simulink model "LinearesSystem"  (R2021b)
settings: Solver=ode4  StartTime=0.0  StopTime=50  FixedStep=0.02  RelTol=1e-3
undefined symbols (not defined in the file): BFZ, ENV
settings Model: Creator=jonih  LastModifiedBy=jonih

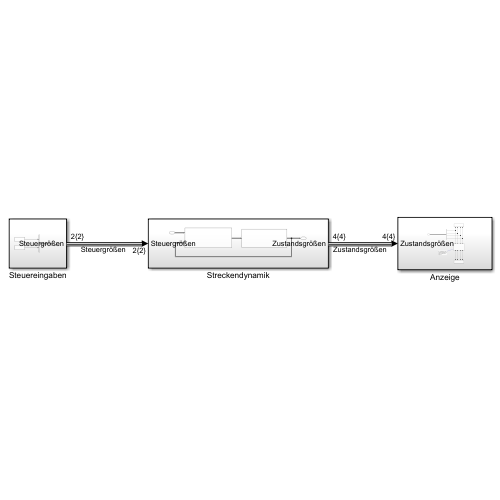
[thumbnail: Simulink's stored preview of the top-level diagram]
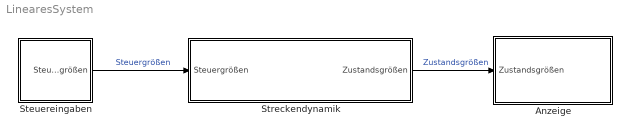
== system LinearesSystem ==
  Anzeige : Subsystem
  Steuereingaben : Subsystem
  Streckendynamik : Subsystem
  wires:
  Steuereingaben/1(Steuergrößen) -> Streckendynamik/1(Steuergrößen)  "Steuergrößen"
  Streckendynamik/1(Zustandsgrößen) -> Anzeige/1(Zustandsgrößen)  "Zustandsgrößen"

== system LinearesSystem/Anzeige ==
  note: zur Herstellung der
      | Vergleichbarkeit mit
      | dem nichtlinearen
      | System
  Zustandsgrößen : Inport
  Aufaddierung der Initalwerte : Subsystem
  Bus Selector : BusSelector  OutputSignals=ΔV,Δγ,Δq,Δα
  lineares System : Scope  NumInputPorts=4
  lineares System (angepasst) : Scope  NumInputPorts=4
  wires:
  Zustandsgrößen/1 -> Bus Selector/1  "Abweichung Zust. vom BFZ"
  Bus Selector/1 -> Aufaddierung der Initalwerte/1(<ΔV>), lineares System/1  "<ΔV>"
  Bus Selector/2 -> Aufaddierung der Initalwerte/2(<Δγ>), lineares System/2  "<Δγ>"
  Bus Selector/3 -> lineares System/3, Aufaddierung der Initalwerte/3(<Δq>)  "<Δq>"
  Bus Selector/4 -> lineares System/4, Aufaddierung der Initalwerte/4(<Δα>)  "<Δα>"
  Aufaddierung der Initalwerte/1(V) -> lineares System (angepasst)/1  "V"
  Aufaddierung der Initalwerte/2(gamma) -> lineares System (angepasst)/2  "gamma"
  Aufaddierung der Initalwerte/3(q) -> lineares System (angepasst)/3  "q"
  Aufaddierung der Initalwerte/4(alpha) -> lineares System (angepasst)/4  "alpha"

== system LinearesSystem/Steuereingaben ==
  Bus Creator : BusCreator  Inputs=2
  Δδ : Constant  Value=0
  Δη : Constant  Value=0
  Steuergrößen : Outport
  wires:
  Δη/1 -> Bus Creator/1  "Δη"
  Δδ/1 -> Bus Creator/2  "Δδ"
  Bus Creator/1 -> Steuergrößen/1  "Steuergrößen"

== system LinearesSystem/Streckendynamik ==
  Steuergrößen : Inport
  Berechnung Änderung der Zustandsgrößen : Subsystem
  Integration : Subsystem
  Zustandsgrößen : Outport
  wires:
  Berechnung Änderung der Zustandsgrößen/1(zeitliche Änderung der Zustandsgrößen) -> Integration/1(zeitliche Änderung der Zustandsgrößen)
  Integration/1(Zustandsgrößen) -> Berechnung Änderung der Zustandsgrößen/2(Zustandsgrößen), Zustandsgrößen/1  "Zustandsgrößen"
  Steuergrößen/1 -> Berechnung Änderung der Zustandsgrößen/1(Steuergrößen)

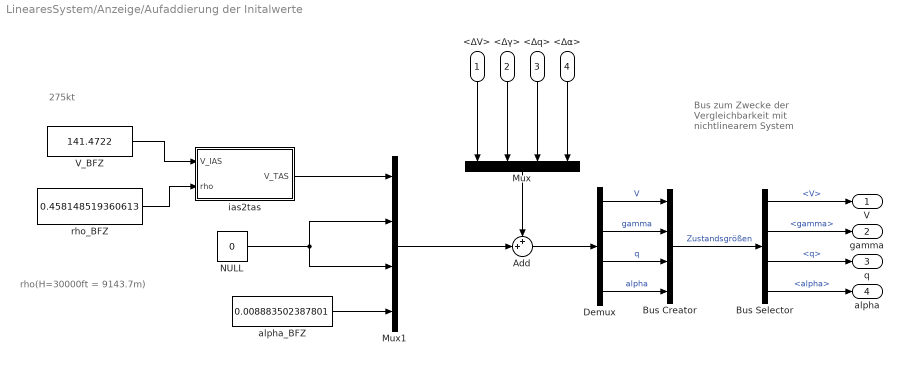
== system LinearesSystem/Anzeige/Aufaddierung der Initalwerte ==
  note: rho(H=30000ft
      | = 9143.7m)
  note: Bus zum Zwecke der
      | Vergleichbarkeit mit
      | nichtlinearem System
  note: 275kt
  <ΔV> : Inport
  <Δγ> : Inport  Port=2
  <Δq> : Inport  Port=3
  <Δα> : Inport  Port=4
  Add : Sum  Inputs=++|
  Bus Creator : BusCreator  Inputs=4
  Bus Selector : BusSelector  OutputSignals=V,gamma,q,alpha
  Demux : Demux
  Mux : Mux
  Mux1 : Mux
  NULL : Constant  Value=0
  V_BFZ : Constant  Value=141.4722
  alpha_BFZ : Constant  Value=0.008883502387801
  ias2tas : Subsystem
  rho_BFZ : Constant  Value=0.458148519360613
  V : Outport
  gamma : Outport  Port=2
  q : Outport  Port=3
  alpha : Outport  Port=4
  wires:
  alpha_BFZ/1 -> Mux1/4
  <Δq>/1 -> Mux/3
  NULL/1 -> Mux1/3, Mux1/2
  <Δα>/1 -> Mux/4
  Add/1 -> Demux/1
  <ΔV>/1 -> Mux/1
  <Δγ>/1 -> Mux/2
  Mux/1 -> Add/1
  Mux1/1 -> Add/2
  Bus Creator/1 -> Bus Selector/1  "Zustandsgrößen"
  Demux/1 -> Bus Creator/1  "V"
  Demux/2 -> Bus Creator/2  "gamma"
  Demux/3 -> Bus Creator/3  "q"
  Demux/4 -> Bus Creator/4  "alpha"
  Bus Selector/1 -> V/1  "<V>"
  Bus Selector/2 -> gamma/1  "<gamma>"
  Bus Selector/3 -> q/1  "<q>"
  Bus Selector/4 -> alpha/1  "<alpha>"
  ias2tas/1(V_TAS) -> Mux1/1
  V_BFZ/1 -> ias2tas/1(V_IAS)
  rho_BFZ/1 -> ias2tas/2(rho)

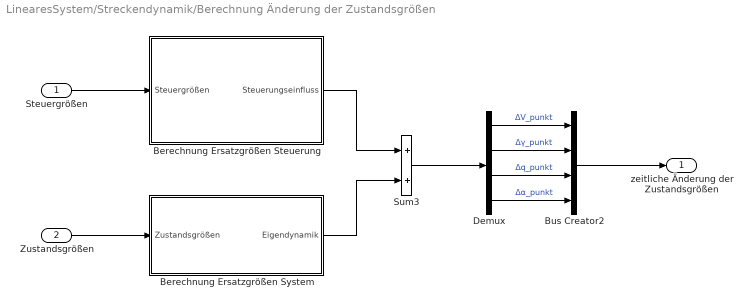
== system LinearesSystem/Streckendynamik/Berechnung Änderung der Zustandsgrößen ==
  Steuergrößen : Inport
  Zustandsgrößen : Inport  Port=2
  Berechnung Ersatzgrößen Steuerung : Subsystem
  Berechnung Ersatzgrößen System : Subsystem
  Bus Creator2 : BusCreator  Inputs=4
  Demux : Demux
  Sum3 : Sum
  zeitliche Änderung der Zustandsgrößen : Outport
  wires:
  Demux/4 -> Bus Creator2/4  "Δα_punkt"
  Demux/2 -> Bus Creator2/2  "Δγ_punkt"
  Demux/3 -> Bus Creator2/3  "Δq_punkt"
  Demux/1 -> Bus Creator2/1  "ΔV_punkt"
  Zustandsgrößen/1 -> Berechnung Ersatzgrößen System/1(Zustandsgrößen)
  Bus Creator2/1 -> zeitliche Änderung der Zustandsgrößen/1
  Steuergrößen/1 -> Berechnung Ersatzgrößen Steuerung/1(Steuergrößen)
  Sum3/1 -> Demux/1
  Berechnung Ersatzgrößen Steuerung/1(Steuerungseinfluss) -> Sum3/1
  Berechnung Ersatzgrößen System/1(Eigendynamik) -> Sum3/2

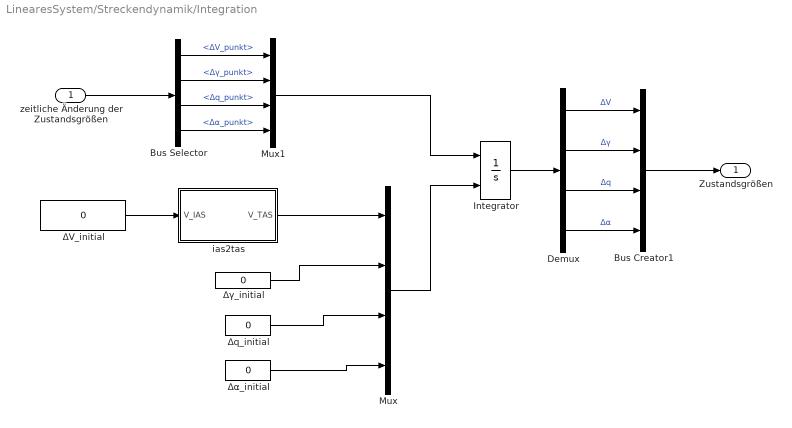
== system LinearesSystem/Streckendynamik/Integration ==
  zeitliche Änderung der Zustandsgrößen : Inport
  Bus Creator1 : BusCreator  Inputs=4
  Bus Selector : BusSelector  OutputSignals=ΔV_punkt,Δγ_punkt,Δq_punkt,Δα_punkt
  Demux : Demux
  Integrator : Integrator  InitialConditionSource=external
  Mux : Mux
  Mux1 : Mux
  ias2tas : Subsystem
  ΔV_initial : Constant  Value=0
  Δq_initial : Constant  Value=0
  Δα_initial : Constant  Value=0
  Δγ_initial : Constant  Value=0
  Zustandsgrößen : Outport
  wires:
  zeitliche Änderung der Zustandsgrößen/1 -> Bus Selector/1
  Δγ_initial/1 -> Mux/2
  Δα_initial/1 -> Mux/4
  Δq_initial/1 -> Mux/3
  Bus Creator1/1 -> Zustandsgrößen/1
  ias2tas/1(V_TAS) -> Mux/1
  Mux1/1 -> Integrator/1
  Bus Selector/1 -> Mux1/1  "<ΔV_punkt>"
  Bus Selector/2 -> Mux1/2  "<Δγ_punkt>"
  Bus Selector/3 -> Mux1/3  "<Δq_punkt>"
  Bus Selector/4 -> Mux1/4  "<Δα_punkt>"
  Mux/1 -> Integrator/2
  Demux/1 -> Bus Creator1/1  "ΔV"
  Demux/2 -> Bus Creator1/2  "Δγ"
  Demux/3 -> Bus Creator1/3  "Δq"
  Demux/4 -> Bus Creator1/4  "Δα"
  Integrator/1 -> Demux/1
  ΔV_initial/1 -> ias2tas/1(V_IAS)

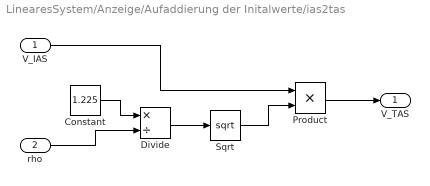
== system LinearesSystem/Anzeige/Aufaddierung der Initalwerte/ias2tas ==
  V_IAS : Inport
  rho : Inport  Port=2
  Constant : Constant  Value=1.225
  Divide : Product  Inputs=*/
  Product : Product
  Sqrt : Sqrt  SaturateOnIntegerOverflow=on
  V_TAS : Outport
  wires:
  Product/1 -> V_TAS/1
  V_IAS/1 -> Product/1
  Constant/1 -> Divide/1
  rho/1 -> Divide/2
  Divide/1 -> Sqrt/1
  Sqrt/1 -> Product/2

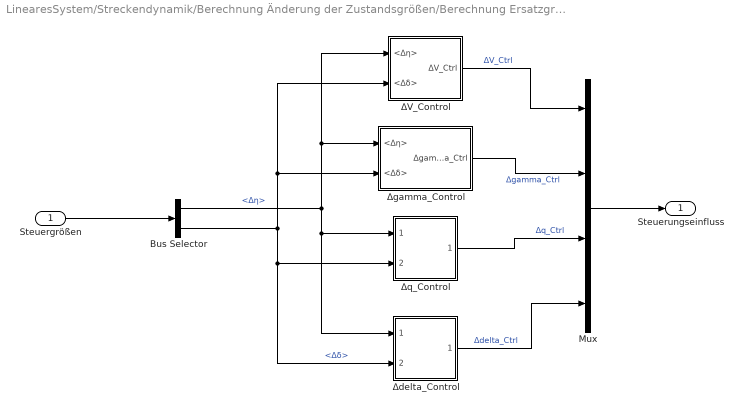
== system LinearesSystem/Streckendynamik/Berechnung Änderung der Zustandsgrößen/Berechnung Ersatzgrößen Steuerung ==
  Steuergrößen : Inport
  Bus Selector : BusSelector  OutputSignals=Δη,Δδ
  Mux : Mux
  ΔV_Control : Subsystem
  Δdelta_Control : Subsystem
  Δgamma_Control : Subsystem
  Δq_Control : Subsystem
  Steuerungseinfluss : Outport
  wires:
  Bus Selector/2 -> Δdelta_Control/2(<Δδ>), Δq_Control/2(<Δδ>), Δgamma_Control/2(<Δδ>), ΔV_Control/2(<Δδ>)  "<Δδ>"
  Steuergrößen/1 -> Bus Selector/1
  Bus Selector/1 -> Δq_Control/1(<Δη>), Δdelta_Control/1(<Δη>), Δgamma_Control/1(<Δη>), ΔV_Control/1(<Δη>)  "<Δη>"
  ΔV_Control/1(ΔV_Ctrl) -> Mux/1  "ΔV_Ctrl"
  Δgamma_Control/1(Δgamma_Ctrl) -> Mux/2  "Δgamma_Ctrl"
  Δq_Control/1(Δq_Ctrl) -> Mux/3  "Δq_Ctrl"
  Δdelta_Control/1(Δdelta_Ctrl) -> Mux/4  "Δdelta_Ctrl"
  Mux/1 -> Steuerungseinfluss/1

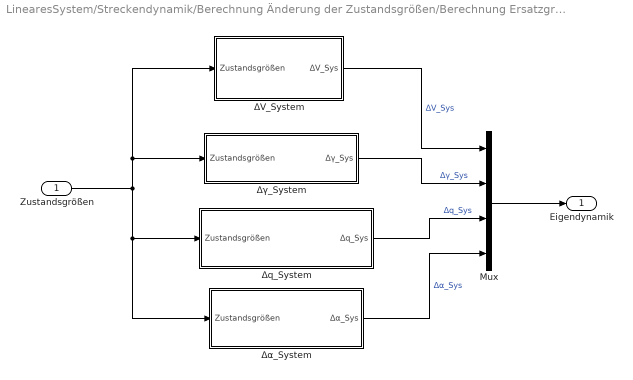
== system LinearesSystem/Streckendynamik/Berechnung Änderung der Zustandsgrößen/Berechnung Ersatzgrößen System ==
  Zustandsgrößen : Inport
  Mux : Mux
  ΔV_System : Subsystem
  Δq_System : Subsystem
  Δα_System : Subsystem
  Δγ_System : Subsystem
  Eigendynamik : Outport
  wires:
  Δγ_System/1(Δγ_Sys) -> Mux/2  "Δγ_Sys"
  Zustandsgrößen/1 -> Δγ_System/1(Zustandsgrößen), ΔV_System/1(Zustandsgrößen), Δq_System/1(Zustandsgrößen), Δα_System/1(Zustandsgrößen)
  Δα_System/1(Δα_Sys) -> Mux/4  "Δα_Sys"
  Δq_System/1(Δq_Sys) -> Mux/3  "Δq_Sys"
  ΔV_System/1(ΔV_Sys) -> Mux/1  "ΔV_Sys"
  Mux/1 -> Eigendynamik/1

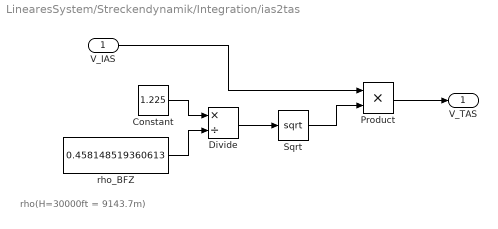
== system LinearesSystem/Streckendynamik/Integration/ias2tas ==
  note: rho(H=30000ft
      | = 9143.7m)
  V_IAS : Inport
  Constant : Constant  Value=1.225
  Divide : Product  Inputs=*/
  Product : Product
  Sqrt : Sqrt  SaturateOnIntegerOverflow=on
  rho_BFZ : Constant  Value=0.458148519360613
  V_TAS : Outport
  wires:
  Product/1 -> V_TAS/1
  V_IAS/1 -> Product/1
  Constant/1 -> Divide/1
  Divide/1 -> Sqrt/1
  Sqrt/1 -> Product/2
  rho_BFZ/1 -> Divide/2

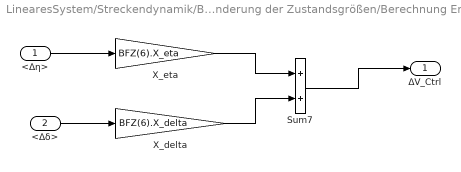
== system LinearesSystem/Streckendynamik/Berechnung Änderung der Zustandsgrößen/Berechnung Ersatzgrößen Steuerung/ΔV_Control ==
  <Δη> : Inport
  <Δδ> : Inport  Port=2
  Sum7 : Sum
  X_delta : Gain  Gain=BFZ(6).X_delta
  X_eta : Gain  Gain=BFZ(6).X_eta
  ΔV_Ctrl : Outport
  wires:
  X_eta/1 -> Sum7/1
  <Δδ>/1 -> X_delta/1
  X_delta/1 -> Sum7/2
  <Δη>/1 -> X_eta/1
  Sum7/1 -> ΔV_Ctrl/1

== system LinearesSystem/Streckendynamik/Berechnung Änderung der Zustandsgrößen/Berechnung Ersatzgrößen Steuerung/Δdelta_Control ==
  <Δη> : Inport
  <Δδ> : Inport  Port=2
  Sum4 : Sum
  Z_delta : Gain  Gain=BFZ(6).Z_delta
  Z_eta : Gain  Gain=BFZ(6).Z_eta
  Δdelta_Ctrl : Outport
  wires:
  Z_eta/1 -> Sum4/1
  Z_delta/1 -> Sum4/2
  <Δδ>/1 -> Z_delta/1
  Sum4/1 -> Δdelta_Ctrl/1  "B_4"
  <Δη>/1 -> Z_eta/1

== system LinearesSystem/Streckendynamik/Berechnung Änderung der Zustandsgrößen/Berechnung Ersatzgrößen Steuerung/Δgamma_Control ==
  <Δη> : Inport
  <Δδ> : Inport  Port=2
  Sum8 : Sum  Inputs=--
  Z_delta1 : Gain  Gain=BFZ(6).Z_delta
  Z_eta1 : Gain  Gain=BFZ(6).Z_eta
  Δgamma_Ctrl : Outport
  wires:
  Z_eta1/1 -> Sum8/1
  <Δδ>/1 -> Z_delta1/1
  Z_delta1/1 -> Sum8/2
  <Δη>/1 -> Z_eta1/1
  Sum8/1 -> Δgamma_Ctrl/1  "B_2"

== system LinearesSystem/Streckendynamik/Berechnung Änderung der Zustandsgrößen/Berechnung Ersatzgrößen Steuerung/Δq_Control ==
  <Δη> : Inport
  <Δδ> : Inport  Port=2
  M_delta : Gain  Gain=BFZ(6).M_delta
  M_eta : Gain  Gain=BFZ(6).M_eta
  Sum : Sum
  Δq_Ctrl : Outport
  wires:
  <Δδ>/1 -> M_delta/1
  M_eta/1 -> Sum/1
  M_delta/1 -> Sum/2
  Sum/1 -> Δq_Ctrl/1  "B_3"
  <Δη>/1 -> M_eta/1

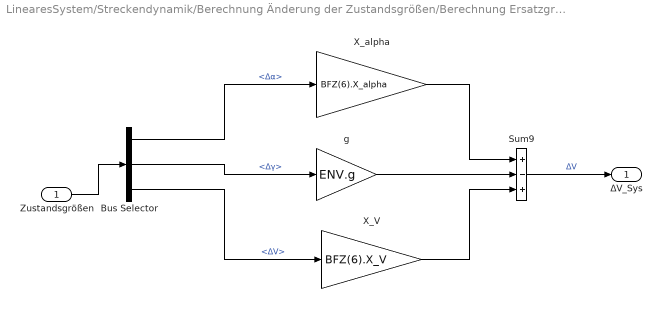
== system LinearesSystem/Streckendynamik/Berechnung Änderung der Zustandsgrößen/Berechnung Ersatzgrößen System/ΔV_System ==
  Zustandsgrößen : Inport
  Bus Selector : BusSelector  OutputSignals=Δα,Δγ,ΔV
  Sum9 : Sum  Inputs=+-+
  X_V : Gain  Gain=BFZ(6).X_V
  X_alpha : Gain  Gain=BFZ(6).X_alpha
  g : Gain  Gain=ENV.g
  ΔV_Sys : Outport
  wires:
  Bus Selector/1 -> X_alpha/1  "<Δα>"
  Sum9/1 -> ΔV_Sys/1  "ΔV"
  g/1 -> Sum9/2
  Zustandsgrößen/1 -> Bus Selector/1
  X_V/1 -> Sum9/3
  X_alpha/1 -> Sum9/1
  Bus Selector/2 -> g/1  "<Δγ>"
  Bus Selector/3 -> X_V/1  "<ΔV>"

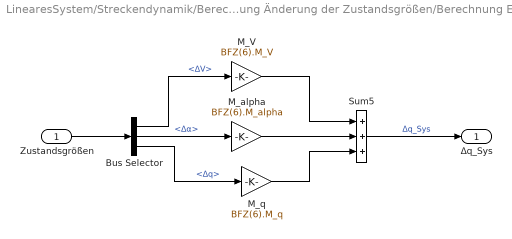
== system LinearesSystem/Streckendynamik/Berechnung Änderung der Zustandsgrößen/Berechnung Ersatzgrößen System/Δq_System ==
  Zustandsgrößen : Inport
  Bus Selector : BusSelector  OutputSignals=ΔV,Δα,Δq
  M_V : Gain  Gain=BFZ(6).M_V
  M_alpha : Gain  Gain=BFZ(6).M_alpha
  M_q : Gain  Gain=BFZ(6).M_q
  Sum5 : Sum  Inputs=+++
  Δq_Sys : Outport
  wires:
  Bus Selector/2 -> M_alpha/1  "<Δα>"
  Bus Selector/1 -> M_V/1  "<ΔV>"
  Sum5/1 -> Δq_Sys/1  "Δq_Sys"
  Bus Selector/3 -> M_q/1  "<Δq>"
  Zustandsgrößen/1 -> Bus Selector/1
  M_alpha/1 -> Sum5/2
  M_V/1 -> Sum5/1
  M_q/1 -> Sum5/3

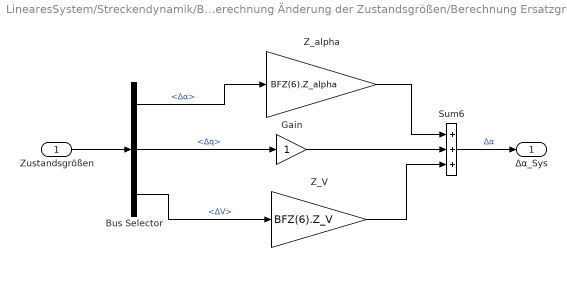
== system LinearesSystem/Streckendynamik/Berechnung Änderung der Zustandsgrößen/Berechnung Ersatzgrößen System/Δα_System ==
  Zustandsgrößen : Inport
  Bus Selector : BusSelector  OutputSignals=Δα,Δq,ΔV
  Gain : Gain
  Sum6 : Sum  Inputs=+++
  Z_V : Gain  Gain=BFZ(6).Z_V
  Z_alpha : Gain  Gain=BFZ(6).Z_alpha
  Δα_Sys : Outport
  wires:
  Bus Selector/1 -> Z_alpha/1  "<Δα>"
  Bus Selector/2 -> Gain/1  "<Δq>"
  Bus Selector/3 -> Z_V/1  "<ΔV>"
  Sum6/1 -> Δα_Sys/1  "Δα"
  Z_alpha/1 -> Sum6/1
  Gain/1 -> Sum6/2
  Z_V/1 -> Sum6/3
  Zustandsgrößen/1 -> Bus Selector/1

== system LinearesSystem/Streckendynamik/Berechnung Änderung der Zustandsgrößen/Berechnung Ersatzgrößen System/Δγ_System ==
  Zustandsgrößen : Inport
  Bus Selector : BusSelector  OutputSignals=Δα,ΔV
  Sum2 : Sum  Inputs=--
  Z_V : Gain  Gain=BFZ(6).Z_V
  Z_alpha : Gain  Gain=BFZ(6).Z_alpha
  Δγ_Sys : Outport
  wires:
  Bus Selector/2 -> Z_V/1  "<ΔV>"
  Bus Selector/1 -> Z_alpha/1  "<Δα>"
  Sum2/1 -> Δγ_Sys/1  "Δγ"
  Zustandsgrößen/1 -> Bus Selector/1
  Z_alpha/1 -> Sum2/1
  Z_V/1 -> Sum2/2
